simulink library "HybridMpcLib"  (Simulink 7.8)
settings: Solver=ode45  StartTime=0.0  StopTime=10.0  RelTol=1e-3
values from neighbouring files (symbols this model uses):
  A = [0  1       0 ... (first row only)    [TTR_KA.m]    (also in mpt3pwacplextst.mat = [0 0 0 0 1 -0.1 0 0 0 0 0 0 ... (16 elements, 4x4)]; tmp_wrkspc.mat = [0  1  0; 0  -0.1  9.16460526316; 0  0  -4.63284688441]; ttrx.m = [0  1)
  B = [0 ... (first row only)    [TTR_KA.m]    (also in mpt3pwacplextst.mat = [0  0; -9.16460526316  0.0738928415604; 0  0; -1.61596717544; tmp_wrkspc.mat = [0 0 4.62121843873]; ttrx.m)
  Fi = cell(nr,1)    [GetMPCMatrices_vP.m]    (also in GetRobustMPCMatrices.m = sol_mp.Fi; GetRobustMPC_Matrices_bk.m = sol_mp.Fi; tmp_wrkspc.mat = )
  Gi = Fi    [GetMPCMatrices_vP.m]    (also in GetRobustMPCMatrices.m = sol_mp.Gi; GetRobustMPC_Matrices_bk.m = sol_mp.Gi; tmp_wrkspc.mat = )
  Hn = {Hn}    [GetMPCMatrices_vP.m]    (also in GetRobustMPCMatrices.m; GetRobustMPC_Matrices_bk.m; tmp_wrkspc.mat = )
  Kn = {Kn}    [GetMPCMatrices_vP.m]    (also in GetRobustMPCMatrices.m; GetRobustMPC_Matrices_bk.m; tmp_wrkspc.mat = )
  Nc = zeros(nr,1)    [GetMPCMatrices_vP.m]    (also in GetRobustMPCMatrices.m; GetRobustMPC_Matrices_bk.m; mpt3pwacplextst.mat = [14 11 10 9 8 12 8 16 15 16 14 9 ... (497 elements, 497x1)]; tmp_wrkspc.mat = [1 1 1 1 1 1 1 1 1 1 1 1 ... (234 elements, 234x1)])
  Ts = 0.01    [mpt3pwacplextst.mat]    (also in tmp_wrkspc.mat = 0.25)
undefined symbols (not defined in the file or in its folder): model, x_init
settings Model: Creator=burrimi  LastModifiedBy=burrimi

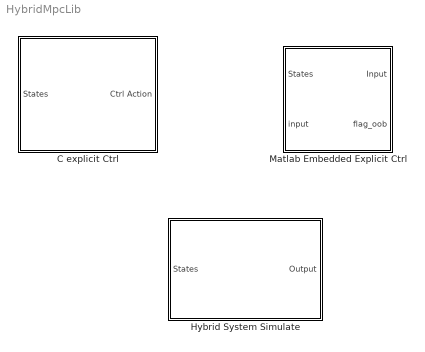
== system HybridMpcLib ==
  C explicit Ctrl : Subsystem
  Hybrid System Simulate : Subsystem
  Matlab Embedded Explicit Ctrl : Subsystem

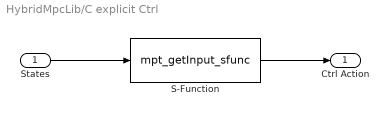
== system HybridMpcLib/C explicit Ctrl ==
  States : Inport
  S-Function : S-Function  FunctionName=mpt_getInput_sfunc  EnableBusSupport=off
  Ctrl Action : Outport
  wires:
  S-Function/1 -> Ctrl Action/1
  States/1 -> S-Function/1

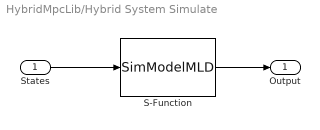
== system HybridMpcLib/Hybrid System Simulate ==
  States : Inport
  S-Function : S-Function  FunctionName=SimModelMLD  Parameters=model,x_init,Ts  EnableBusSupport=off
  Output : Outport
  wires:
  States/1 -> S-Function/1
  S-Function/1 -> Output/1

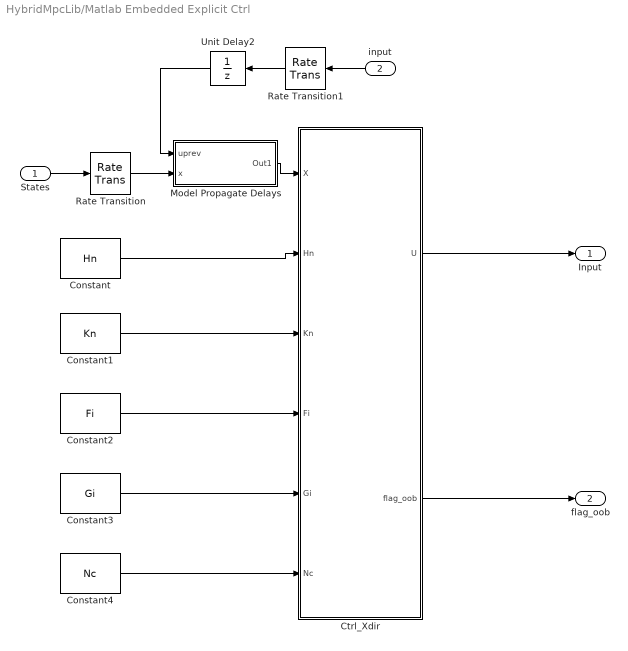
== system HybridMpcLib/Matlab Embedded Explicit Ctrl ==
  States : Inport
  input : Inport  Port=2
  Constant : Constant  Value=Hn
  Constant1 : Constant  Value=Kn
  Constant2 : Constant  Value=Fi
  Constant3 : Constant  Value=Gi
  Constant4 : Constant  Value=Nc
  Ctrl_Xdir : MATLAB Function  TreatAsAtomicUnit=on
  Model Propagate Delays : Subsystem
  Rate Transition : RateTransition  OutPortSampleTime=TsCtrl
  Rate Transition1 : RateTransition  OutPortSampleTime=TsCtrl
  Unit Delay2 : UnitDelay  SampleTime=-1
  Input : Outport
  flag_oob : Outport  Port=2
  wires:
  Ctrl_Xdir/2(flag_oob) -> flag_oob/1
  Ctrl_Xdir/1(U) -> Input/1
  Constant4/1 -> Ctrl_Xdir/6(Nc)
  Constant3/1 -> Ctrl_Xdir/5(Gi)
  Constant2/1 -> Ctrl_Xdir/4(Fi)
  Constant1/1 -> Ctrl_Xdir/3(Kn)
  Constant/1 -> Ctrl_Xdir/2(Hn)
  States/1 -> Rate Transition/1
  Unit Delay2/1 -> Model Propagate Delays/1(uprev)
  Rate Transition/1 -> Model Propagate Delays/2(x)
  Model Propagate Delays/1(Out1) -> Ctrl_Xdir/1(X)
  input/1 -> Rate Transition1/1
  Rate Transition1/1 -> Unit Delay2/1

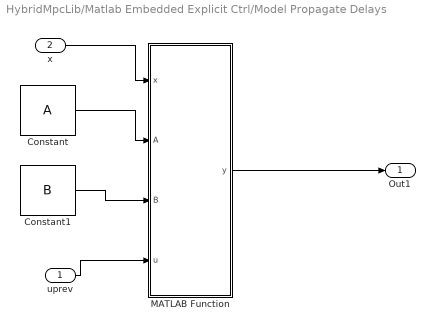
== system HybridMpcLib/Matlab Embedded Explicit Ctrl/Model Propagate Delays ==
  uprev : Inport
  x : Inport  Port=2
  Constant : Constant  Value=A
  Constant1 : Constant  Value=B
  MATLAB Function : MATLAB Function  TreatAsAtomicUnit=on
  Out1 : Outport
  wires:
  MATLAB Function/1(y) -> Out1/1
  x/1 -> MATLAB Function/1(x)
  uprev/1 -> MATLAB Function/4(u)
  Constant/1 -> MATLAB Function/2(A)
  Constant1/1 -> MATLAB Function/3(B)

== matlab function Matlab Embedded Explicit Ctrl/Ctrl_Xdir ==
  data: X input double; U output double; Hn input double; Kn input double; Fi input double; Gi input double; Nc input double; flag_oob output double
function [U,flag_oob] = OptimalMPCInput(X,Hn,Kn,Fi,Gi,Nc)

tolerance = 1;
nr  = size(Nc,1);
MPT_ABSTOL = 1e-8;
minreg = 0;
X = round(10000*X)/10000;

flag_oob = 0;
%maxSize = max(Nc);

Hi = zeros(1000,4);
Ki = zeros(1000,1);

% Find the proper region
abspos = 1;
for ireg = 1:nr
    sumViol = 0;
    isinside = 1;
    

  %  Hi(1:Nc(ireg),1:4) = Hn(abspos:(abspos+Nc(ireg)-1),1:4);
    for i = 1:Nc(ireg)
        for j = 1:4
            Hi(i,j) = Hn(abspos + i - 1,j);
        end
    end
    
%    Ki(1:Nc(ireg),1) = Kn(abspos:(abspos+Nc(ireg)-1),1);
    for i = 1:Nc(ireg)
        Ki(i,1) = Kn(abspos + i - 1,1);
    end
    abspos = abspos + Nc(ireg);
    
    F = Fi(ireg,:);
    G = Gi(ireg,:);
    
    nc = Nc(ireg);
    
    for ic = 1:nc
        hx = Hi(ic,:)*X;
        if ((hx - Ki(ic)) > MPT_ABSTOL)
            isinside = 0;
            sumViol = sumViol + (hx - Ki(ic));
        end
    end
    
    if (sumViol < tolerance)
        tolerance = sumViol;
        minreg = ireg;
    end
    % extract the right control law
    if (isinside == 1)
        U = F*X + G;
        return
    end
end
F = Fi(minreg,:);
G = Gi(minreg,:);
U = F*X + G;
flag_oob = 1;
return

== matlab function Matlab Embedded Explicit Ctrl/Model Propagate Delays/MATLAB Function ==
  data: x input double; y output double; A input double; B input double; u input double
function y = fcn(x,A,B,u)
%#codegen

y = A*x + B*u;
